simulink library "Computer_Library"  (Simulink 8.1)
settings: Solver=ode45  StartTime=0.0  StopTime=10.0  RelTol=1e-3
values from neighbouring files (symbols this model uses):
  A = 10    [CharTable.m]
  ARROW_DOWN = 48    [CharTable.m]
  ARROW_LEFT = 49    [CharTable.m]
  ARROW_RIGHT = 50    [CharTable.m]
  ARROW_UP = 47    [CharTable.m]
  ASTERISK = 39    [CharTable.m]
  B = 11    [CharTable.m]
  BACKSLASH = 43    [CharTable.m]
  C = 12    [CharTable.m]
  COLON = 40    [CharTable.m]
  COMMA = 53    [CharTable.m]
  CROSS = 38    [CharTable.m]
  CURSOR = 62    [CharTable.m]
  D = 13    [CharTable.m]
  DOT = 52    [CharTable.m]
  EQUAL = 44    [CharTable.m]
  EXCLAMATION_MARK = 55    [CharTable.m]
  F = 15    [CharTable.m]
  G = 16    [CharTable.m]
  GREATER_THAN = 46    [CharTable.m]
  H = 17    [CharTable.m]
  I = 18    [CharTable.m]
  J = 19    [CharTable.m]
  K = 20    [CharTable.m]
  L = 21    [CharTable.m]
  LEFT_PARENTHESES = 59    [CharTable.m]
  LESS_THAN = 45    [CharTable.m]
  M = 22    [CharTable.m]
  MINUS = 37    [CharTable.m]
  N = 23    [CharTable.m]
  O = 24    [CharTable.m]
  P = 25    [CharTable.m]
  PERCENT = 58    [CharTable.m]
  PLUS = 36    [CharTable.m]
  Q = 32    [CharTable.m]
  QUESTION_MARK = 54    [CharTable.m]
  QUOTE = 56    [CharTable.m]
  R = 26    [CharTable.m]
  RECTANGLE = 63    [CharTable.m]
  RIGHT_PARENTHESES = 60    [CharTable.m]
  RomCode = reshape(transpose(RomCode), [], 1)    [ROM.m]
  S = 27    [CharTable.m]
  SEMICOLON = 41    [CharTable.m]
  SHARP = 57    [CharTable.m]
  SLASH = 42    [CharTable.m]
  SPACE = 61    [CharTable.m]
  T = 28    [CharTable.m]
  U = 29    [CharTable.m]
  UNDERSCORE = 51    [CharTable.m]
  V = 30    [CharTable.m]
  W = 31    [CharTable.m]
  X = 33    [CharTable.m]
  Y = 34    [CharTable.m]
  Z = 35    [CharTable.m]
undefined symbols (not defined in the file or in its folder): char_0
libraries: Memory_Blocks_Lib x116, Byte_Multiplexers_Lib x44, commutil2 x18, Bit_Multiplexers_Lib x17, Decoders_Lib x9, simulink_extras x8, Logic_Operations_Lib x4, Byte_Demultiplexers_Lib x2, Arithmetic_Operations_Lib x2, dspsnks4 x1
(part 3 of 4)

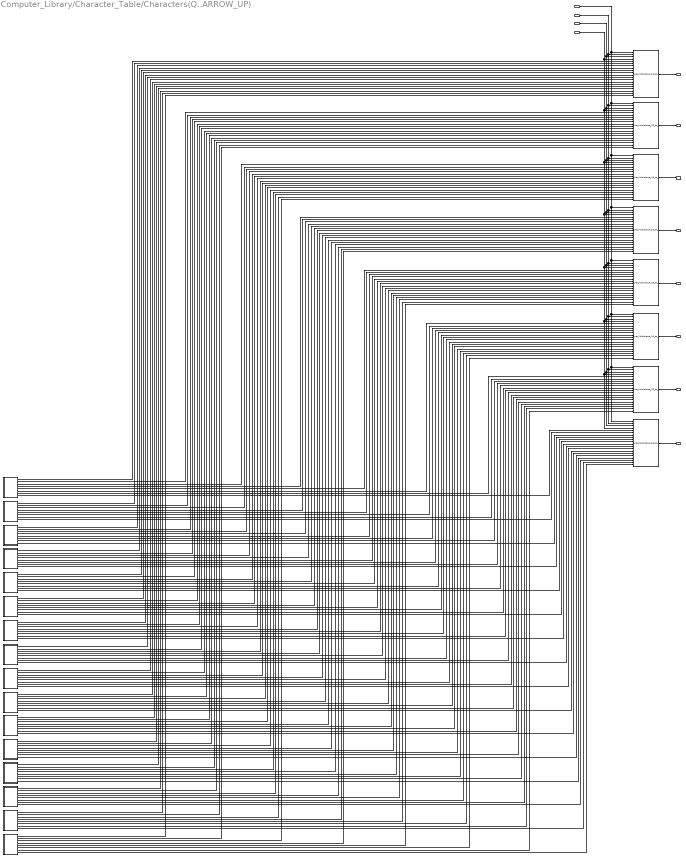
== system Computer_Library/Character_Table/Characters(Q..ARROW_UP) ==
  Address_3_In(1b) : Inport
  Address_2_In(1b) : Inport  Port=2
  Address_1_In(1b) : Inport  Port=3
  Address_0_In(1b) : Inport  Port=4
  16_to_1_Byte_Multiplexer{,1..7} (8 alike) : Byte_Multiplexers_Lib/Byte_Multiplexers_Lib/Byte_Multiplexer_16_to_1
  Char_ARROW_UP : Subsystem
  Char_ASTERISK : Subsystem
  Char_BACKSLASH : Subsystem
  Char_COLON : Subsystem
  Char_CROSS : Subsystem
  Char_EQUAL : Subsystem
  Char_GREATER_THAN : Subsystem
  Char_LESS_THAN : Subsystem
  Char_MINUS : Subsystem
  Char_PLUS : Subsystem
  Char_Q : Subsystem
  Char_SEMICOLON : Subsystem
  Char_SLASH : Subsystem
  Char_X : Subsystem
  Char_Y : Subsystem
  Char_Z : Subsystem
  Column_1(1B) : Outport
  Column_2(1B) : Outport  Port=2
  Column_3(1B) : Outport  Port=3
  Column_4(1B) : Outport  Port=4
  Column_5(1B) : Outport  Port=5
  Column_6(1B) : Outport  Port=6
  Column_7(1B) : Outport  Port=7
  Column_8(1B) : Outport  Port=8
  wires:
  Char_ARROW_UP/1(Column_1(1B)) -> 16_to_1_Byte_Multiplexer/5
  Char_GREATER_THAN/1(Column_1(1B)) -> 16_to_1_Byte_Multiplexer/6
  Char_LESS_THAN/1(Column_1(1B)) -> 16_to_1_Byte_Multiplexer/7
  Char_EQUAL/1(Column_1(1B)) -> 16_to_1_Byte_Multiplexer/8
  Char_BACKSLASH/1(Column_1(1B)) -> 16_to_1_Byte_Multiplexer/9
  Char_SLASH/1(Column_1(1B)) -> 16_to_1_Byte_Multiplexer/10
  Char_SEMICOLON/1(Column_1(1B)) -> 16_to_1_Byte_Multiplexer/11
  Char_COLON/1(Column_1(1B)) -> 16_to_1_Byte_Multiplexer/12
  Char_ASTERISK/1(Column_1(1B)) -> 16_to_1_Byte_Multiplexer/13
  Char_CROSS/1(Column_1(1B)) -> 16_to_1_Byte_Multiplexer/14
  Char_MINUS/1(Column_1(1B)) -> 16_to_1_Byte_Multiplexer/15
  Char_PLUS/1(Column_1(1B)) -> 16_to_1_Byte_Multiplexer/16
  Char_Z/1(Column_1(1B)) -> 16_to_1_Byte_Multiplexer/17
  Char_Y/1(Column_1(1B)) -> 16_to_1_Byte_Multiplexer/18
  Char_X/1(Column_1(1B)) -> 16_to_1_Byte_Multiplexer/19
  Char_Q/1(Column_1(1B)) -> 16_to_1_Byte_Multiplexer/20
  Char_ARROW_UP/2(Column_2(1B)) -> 16_to_1_Byte_Multiplexer1/5
  Char_Q/2(Column_2(1B)) -> 16_to_1_Byte_Multiplexer1/20
  Char_X/2(Column_2(1B)) -> 16_to_1_Byte_Multiplexer1/19
  Char_Y/2(Column_2(1B)) -> 16_to_1_Byte_Multiplexer1/18
  Char_Z/2(Column_2(1B)) -> 16_to_1_Byte_Multiplexer1/17
  Char_PLUS/2(Column_2(1B)) -> 16_to_1_Byte_Multiplexer1/16
  Char_MINUS/2(Column_2(1B)) -> 16_to_1_Byte_Multiplexer1/15
  Char_CROSS/2(Column_2(1B)) -> 16_to_1_Byte_Multiplexer1/14
  Char_ASTERISK/2(Column_2(1B)) -> 16_to_1_Byte_Multiplexer1/13
  Char_COLON/2(Column_2(1B)) -> 16_to_1_Byte_Multiplexer1/12
  Char_SEMICOLON/2(Column_2(1B)) -> 16_to_1_Byte_Multiplexer1/11
  Char_SLASH/2(Column_2(1B)) -> 16_to_1_Byte_Multiplexer1/10
  Char_BACKSLASH/2(Column_2(1B)) -> 16_to_1_Byte_Multiplexer1/9
  Char_EQUAL/2(Column_2(1B)) -> 16_to_1_Byte_Multiplexer1/8
  Char_LESS_THAN/2(Column_2(1B)) -> 16_to_1_Byte_Multiplexer1/7
  Char_GREATER_THAN/2(Column_2(1B)) -> 16_to_1_Byte_Multiplexer1/6
  Char_Q/3(Column_3(1B)) -> 16_to_1_Byte_Multiplexer2/20
  Char_X/3(Column_3(1B)) -> 16_to_1_Byte_Multiplexer2/19
  Char_Y/3(Column_3(1B)) -> 16_to_1_Byte_Multiplexer2/18
  Char_Z/3(Column_3(1B)) -> 16_to_1_Byte_Multiplexer2/17
  Char_PLUS/3(Column_3(1B)) -> 16_to_1_Byte_Multiplexer2/16
  Char_MINUS/3(Column_3(1B)) -> 16_to_1_Byte_Multiplexer2/15
  Char_CROSS/3(Column_3(1B)) -> 16_to_1_Byte_Multiplexer2/14
  Char_ASTERISK/3(Column_3(1B)) -> 16_to_1_Byte_Multiplexer2/13
  Char_COLON/3(Column_3(1B)) -> 16_to_1_Byte_Multiplexer2/12
  Char_SEMICOLON/3(Column_3(1B)) -> 16_to_1_Byte_Multiplexer2/11
  Char_SLASH/3(Column_3(1B)) -> 16_to_1_Byte_Multiplexer2/10
  Char_BACKSLASH/3(Column_3(1B)) -> 16_to_1_Byte_Multiplexer2/9
  Char_EQUAL/3(Column_3(1B)) -> 16_to_1_Byte_Multiplexer2/8
  Char_LESS_THAN/3(Column_3(1B)) -> 16_to_1_Byte_Multiplexer2/7
  Char_GREATER_THAN/3(Column_3(1B)) -> 16_to_1_Byte_Multiplexer2/6
  Char_ARROW_UP/3(Column_3(1B)) -> 16_to_1_Byte_Multiplexer2/5
  Char_Q/4(Column_4(1B)) -> 16_to_1_Byte_Multiplexer3/20
  Char_X/4(Column_4(1B)) -> 16_to_1_Byte_Multiplexer3/19
  Char_Y/4(Column_4(1B)) -> 16_to_1_Byte_Multiplexer3/18
  Char_Z/4(Column_4(1B)) -> 16_to_1_Byte_Multiplexer3/17
  Char_PLUS/4(Column_4(1B)) -> 16_to_1_Byte_Multiplexer3/16
  Char_MINUS/4(Column_4(1B)) -> 16_to_1_Byte_Multiplexer3/15
  Char_CROSS/4(Column_4(1B)) -> 16_to_1_Byte_Multiplexer3/14
  Char_ASTERISK/4(Column_4(1B)) -> 16_to_1_Byte_Multiplexer3/13
  Char_COLON/4(Column_4(1B)) -> 16_to_1_Byte_Multiplexer3/12
  Char_SEMICOLON/4(Column_4(1B)) -> 16_to_1_Byte_Multiplexer3/11
  Char_SLASH/4(Column_4(1B)) -> 16_to_1_Byte_Multiplexer3/10
  Char_BACKSLASH/4(Column_4(1B)) -> 16_to_1_Byte_Multiplexer3/9
  Char_EQUAL/4(Column_4(1B)) -> 16_to_1_Byte_Multiplexer3/8
  Char_LESS_THAN/4(Column_4(1B)) -> 16_to_1_Byte_Multiplexer3/7
  Char_GREATER_THAN/4(Column_4(1B)) -> 16_to_1_Byte_Multiplexer3/6
  Char_ARROW_UP/4(Column_4(1B)) -> 16_to_1_Byte_Multiplexer3/5
  Char_Q/5(Column_5(1B)) -> 16_to_1_Byte_Multiplexer4/20
  Char_X/5(Column_5(1B)) -> 16_to_1_Byte_Multiplexer4/19
  Char_Y/5(Column_5(1B)) -> 16_to_1_Byte_Multiplexer4/18
  Char_Z/5(Column_5(1B)) -> 16_to_1_Byte_Multiplexer4/17
  Char_PLUS/5(Column_5(1B)) -> 16_to_1_Byte_Multiplexer4/16
  Char_MINUS/5(Column_5(1B)) -> 16_to_1_Byte_Multiplexer4/15
  Char_ASTERISK/5(Column_5(1B)) -> 16_to_1_Byte_Multiplexer4/13
  Char_CROSS/5(Column_5(1B)) -> 16_to_1_Byte_Multiplexer4/14
  Char_COLON/5(Column_5(1B)) -> 16_to_1_Byte_Multiplexer4/12
  Char_SEMICOLON/5(Column_5(1B)) -> 16_to_1_Byte_Multiplexer4/11
  Char_SLASH/5(Column_5(1B)) -> 16_to_1_Byte_Multiplexer4/10
  Char_BACKSLASH/5(Column_5(1B)) -> 16_to_1_Byte_Multiplexer4/9
  Char_EQUAL/5(Column_5(1B)) -> 16_to_1_Byte_Multiplexer4/8
  Char_LESS_THAN/5(Column_5(1B)) -> 16_to_1_Byte_Multiplexer4/7
  Char_GREATER_THAN/5(Column_5(1B)) -> 16_to_1_Byte_Multiplexer4/6
  Char_ARROW_UP/5(Column_5(1B)) -> 16_to_1_Byte_Multiplexer4/5
  Char_Q/6(Column_6(1B)) -> 16_to_1_Byte_Multiplexer5/20
  Char_X/6(Column_6(1B)) -> 16_to_1_Byte_Multiplexer5/19
  Char_Y/6(Column_6(1B)) -> 16_to_1_Byte_Multiplexer5/18
  Char_Z/6(Column_6(1B)) -> 16_to_1_Byte_Multiplexer5/17
  Char_PLUS/6(Column_6(1B)) -> 16_to_1_Byte_Multiplexer5/16
  Char_MINUS/6(Column_6(1B)) -> 16_to_1_Byte_Multiplexer5/15
  Char_CROSS/6(Column_6(1B)) -> 16_to_1_Byte_Multiplexer5/14
  Char_ASTERISK/6(Column_6(1B)) -> 16_to_1_Byte_Multiplexer5/13
  Char_COLON/6(Column_6(1B)) -> 16_to_1_Byte_Multiplexer5/12
  Char_SEMICOLON/6(Column_6(1B)) -> 16_to_1_Byte_Multiplexer5/11
  Char_SLASH/6(Column_6(1B)) -> 16_to_1_Byte_Multiplexer5/10
  Char_BACKSLASH/6(Column_6(1B)) -> 16_to_1_Byte_Multiplexer5/9
  Char_EQUAL/7(Column_7(1B)) -> 16_to_1_Byte_Multiplexer6/8
  Char_EQUAL/6(Column_6(1B)) -> 16_to_1_Byte_Multiplexer5/8
  Char_LESS_THAN/6(Column_6(1B)) -> 16_to_1_Byte_Multiplexer5/7
  Char_GREATER_THAN/6(Column_6(1B)) -> 16_to_1_Byte_Multiplexer5/6
  Char_ARROW_UP/6(Column_6(1B)) -> 16_to_1_Byte_Multiplexer5/5
  Char_Q/7(Column_7(1B)) -> 16_to_1_Byte_Multiplexer6/20
  Char_X/7(Column_7(1B)) -> 16_to_1_Byte_Multiplexer6/19
  Char_Y/7(Column_7(1B)) -> 16_to_1_Byte_Multiplexer6/18
  Char_Z/7(Column_7(1B)) -> 16_to_1_Byte_Multiplexer6/17
  Char_PLUS/7(Column_7(1B)) -> 16_to_1_Byte_Multiplexer6/16
  Char_MINUS/7(Column_7(1B)) -> 16_to_1_Byte_Multiplexer6/15
  Char_CROSS/7(Column_7(1B)) -> 16_to_1_Byte_Multiplexer6/14
  Char_ASTERISK/7(Column_7(1B)) -> 16_to_1_Byte_Multiplexer6/13
  Char_COLON/7(Column_7(1B)) -> 16_to_1_Byte_Multiplexer6/12
  Char_SEMICOLON/7(Column_7(1B)) -> 16_to_1_Byte_Multiplexer6/11
  Char_SLASH/7(Column_7(1B)) -> 16_to_1_Byte_Multiplexer6/10
  Char_BACKSLASH/7(Column_7(1B)) -> 16_to_1_Byte_Multiplexer6/9
  Char_LESS_THAN/7(Column_7(1B)) -> 16_to_1_Byte_Multiplexer6/7
  Char_GREATER_THAN/7(Column_7(1B)) -> 16_to_1_Byte_Multiplexer6/6
  Char_ARROW_UP/7(Column_7(1B)) -> 16_to_1_Byte_Multiplexer6/5
  Char_Q/8(Column_8(1B)) -> 16_to_1_Byte_Multiplexer7/20
  Char_X/8(Column_8(1B)) -> 16_to_1_Byte_Multiplexer7/19
  Char_Y/8(Column_8(1B)) -> 16_to_1_Byte_Multiplexer7/18
  Char_Z/8(Column_8(1B)) -> 16_to_1_Byte_Multiplexer7/17
  Char_PLUS/8(Column_8(1B)) -> 16_to_1_Byte_Multiplexer7/16
  Char_MINUS/8(Column_8(1B)) -> 16_to_1_Byte_Multiplexer7/15
  Char_CROSS/8(Column_8(1B)) -> 16_to_1_Byte_Multiplexer7/14
  Char_ASTERISK/8(Column_8(1B)) -> 16_to_1_Byte_Multiplexer7/13
  Char_COLON/8(Column_8(1B)) -> 16_to_1_Byte_Multiplexer7/12
  Char_SEMICOLON/8(Column_8(1B)) -> 16_to_1_Byte_Multiplexer7/11
  Char_SLASH/8(Column_8(1B)) -> 16_to_1_Byte_Multiplexer7/10
  Char_BACKSLASH/8(Column_8(1B)) -> 16_to_1_Byte_Multiplexer7/9
  Char_EQUAL/8(Column_8(1B)) -> 16_to_1_Byte_Multiplexer7/8
  Char_LESS_THAN/8(Column_8(1B)) -> 16_to_1_Byte_Multiplexer7/7
  Char_GREATER_THAN/8(Column_8(1B)) -> 16_to_1_Byte_Multiplexer7/6
  Char_ARROW_UP/8(Column_8(1B)) -> 16_to_1_Byte_Multiplexer7/5
  16_to_1_Byte_Multiplexer/1 -> Column_1(1B)/1
  16_to_1_Byte_Multiplexer1/1 -> Column_2(1B)/1
  16_to_1_Byte_Multiplexer2/1 -> Column_3(1B)/1
  16_to_1_Byte_Multiplexer3/1 -> Column_4(1B)/1
  16_to_1_Byte_Multiplexer4/1 -> Column_5(1B)/1
  16_to_1_Byte_Multiplexer5/1 -> Column_6(1B)/1
  16_to_1_Byte_Multiplexer6/1 -> Column_7(1B)/1
  16_to_1_Byte_Multiplexer7/1 -> Column_8(1B)/1
  Address_0_In(1b)/1 -> 16_to_1_Byte_Multiplexer/4, 16_to_1_Byte_Multiplexer1/4, 16_to_1_Byte_Multiplexer2/4, 16_to_1_Byte_Multiplexer3/4, 16_to_1_Byte_Multiplexer4/4, 16_to_1_Byte_Multiplexer5/4, 16_to_1_Byte_Multiplexer6/4, 16_to_1_Byte_Multiplexer7/4
  Address_1_In(1b)/1 -> 16_to_1_Byte_Multiplexer/3, 16_to_1_Byte_Multiplexer1/3, 16_to_1_Byte_Multiplexer2/3, 16_to_1_Byte_Multiplexer3/3, 16_to_1_Byte_Multiplexer4/3, 16_to_1_Byte_Multiplexer5/3, 16_to_1_Byte_Multiplexer6/3, 16_to_1_Byte_Multiplexer7/3
  Address_2_In(1b)/1 -> 16_to_1_Byte_Multiplexer/2, 16_to_1_Byte_Multiplexer1/2, 16_to_1_Byte_Multiplexer2/2, 16_to_1_Byte_Multiplexer3/2, 16_to_1_Byte_Multiplexer4/2, 16_to_1_Byte_Multiplexer5/2, 16_to_1_Byte_Multiplexer6/2, 16_to_1_Byte_Multiplexer7/2
  Address_3_In(1b)/1 -> 16_to_1_Byte_Multiplexer/1, 16_to_1_Byte_Multiplexer1/1, 16_to_1_Byte_Multiplexer2/1, 16_to_1_Byte_Multiplexer3/1, 16_to_1_Byte_Multiplexer4/1, 16_to_1_Byte_Multiplexer5/1, 16_to_1_Byte_Multiplexer6/1, 16_to_1_Byte_Multiplexer7/1

== system Computer_Library/Instruction_ADD/Full_Adder ==
  A : Inport
  B : Inport  Port=2
  Carry_In : Inport  Port=3
  Logical Operator : Logic  Operator=XOR  IconShape=distinctive  AllPortsSameDT=off  OutDataTypeStr=boolean
  Logical Operator1 : Logic  IconShape=distinctive  AllPortsSameDT=off  OutDataTypeStr=boolean
  Logical Operator2 : Logic  Operator=XOR  IconShape=distinctive  AllPortsSameDT=off  OutDataTypeStr=boolean
  Logical Operator3 : Logic  IconShape=distinctive  AllPortsSameDT=off  OutDataTypeStr=boolean
  Logical Operator4 : Logic  Operator=OR  IconShape=distinctive  AllPortsSameDT=off  OutDataTypeStr=boolean
  Carry_Out : Outport
  Sum : Outport  Port=2
  wires:
  A/1 -> Logical Operator1/1, Logical Operator/1
  B/1 -> Logical Operator1/2, Logical Operator/2
  Logical Operator2/1 -> Sum/1
  Logical Operator/1 -> Logical Operator3/1, Logical Operator2/1
  Carry_In/1 -> Logical Operator2/2, Logical Operator3/2
  Logical Operator3/1 -> Logical Operator4/1
  Logical Operator1/1 -> Logical Operator4/2
  Logical Operator4/1 -> Carry_Out/1

== system Computer_Library/Instruction_ADD/Full_Adder1 ==
  A : Inport
  B : Inport  Port=2
  Carry_In : Inport  Port=3
  Logical Operator : Logic  Operator=XOR  IconShape=distinctive  AllPortsSameDT=off  OutDataTypeStr=boolean
  Logical Operator1 : Logic  IconShape=distinctive  AllPortsSameDT=off  OutDataTypeStr=boolean
  Logical Operator2 : Logic  Operator=XOR  IconShape=distinctive  AllPortsSameDT=off  OutDataTypeStr=boolean
  Logical Operator3 : Logic  IconShape=distinctive  AllPortsSameDT=off  OutDataTypeStr=boolean
  Logical Operator4 : Logic  Operator=OR  IconShape=distinctive  AllPortsSameDT=off  OutDataTypeStr=boolean
  Carry_Out : Outport
  Sum : Outport  Port=2
  wires:
  A/1 -> Logical Operator1/1, Logical Operator/1
  B/1 -> Logical Operator1/2, Logical Operator/2
  Logical Operator2/1 -> Sum/1
  Logical Operator/1 -> Logical Operator3/1, Logical Operator2/1
  Carry_In/1 -> Logical Operator2/2, Logical Operator3/2
  Logical Operator3/1 -> Logical Operator4/1
  Logical Operator1/1 -> Logical Operator4/2
  Logical Operator4/1 -> Carry_Out/1

== system Computer_Library/Instruction_ADD/Full_Adder2 ==
  A : Inport
  B : Inport  Port=2
  Carry_In : Inport  Port=3
  Logical Operator : Logic  Operator=XOR  IconShape=distinctive  AllPortsSameDT=off  OutDataTypeStr=boolean
  Logical Operator1 : Logic  IconShape=distinctive  AllPortsSameDT=off  OutDataTypeStr=boolean
  Logical Operator2 : Logic  Operator=XOR  IconShape=distinctive  AllPortsSameDT=off  OutDataTypeStr=boolean
  Logical Operator3 : Logic  IconShape=distinctive  AllPortsSameDT=off  OutDataTypeStr=boolean
  Logical Operator4 : Logic  Operator=OR  IconShape=distinctive  AllPortsSameDT=off  OutDataTypeStr=boolean
  Carry_Out : Outport
  Sum : Outport  Port=2
  wires:
  A/1 -> Logical Operator1/1, Logical Operator/1
  B/1 -> Logical Operator1/2, Logical Operator/2
  Logical Operator2/1 -> Sum/1
  Logical Operator/1 -> Logical Operator3/1, Logical Operator2/1
  Carry_In/1 -> Logical Operator2/2, Logical Operator3/2
  Logical Operator3/1 -> Logical Operator4/1
  Logical Operator1/1 -> Logical Operator4/2
  Logical Operator4/1 -> Carry_Out/1

== system Computer_Library/Instruction_ADD/Full_Adder3 ==
  A : Inport
  B : Inport  Port=2
  Carry_In : Inport  Port=3
  Logical Operator : Logic  Operator=XOR  IconShape=distinctive  AllPortsSameDT=off  OutDataTypeStr=boolean
  Logical Operator1 : Logic  IconShape=distinctive  AllPortsSameDT=off  OutDataTypeStr=boolean
  Logical Operator2 : Logic  Operator=XOR  IconShape=distinctive  AllPortsSameDT=off  OutDataTypeStr=boolean
  Logical Operator3 : Logic  IconShape=distinctive  AllPortsSameDT=off  OutDataTypeStr=boolean
  Logical Operator4 : Logic  Operator=OR  IconShape=distinctive  AllPortsSameDT=off  OutDataTypeStr=boolean
  Carry_Out : Outport
  Sum : Outport  Port=2
  wires:
  A/1 -> Logical Operator1/1, Logical Operator/1
  B/1 -> Logical Operator1/2, Logical Operator/2
  Logical Operator2/1 -> Sum/1
  Logical Operator/1 -> Logical Operator3/1, Logical Operator2/1
  Carry_In/1 -> Logical Operator2/2, Logical Operator3/2
  Logical Operator3/1 -> Logical Operator4/1
  Logical Operator1/1 -> Logical Operator4/2
  Logical Operator4/1 -> Carry_Out/1

== system Computer_Library/Instruction_ADD/Full_Adder4 ==
  A : Inport
  B : Inport  Port=2
  Carry_In : Inport  Port=3
  Logical Operator : Logic  Operator=XOR  IconShape=distinctive  AllPortsSameDT=off  OutDataTypeStr=boolean
  Logical Operator1 : Logic  IconShape=distinctive  AllPortsSameDT=off  OutDataTypeStr=boolean
  Logical Operator2 : Logic  Operator=XOR  IconShape=distinctive  AllPortsSameDT=off  OutDataTypeStr=boolean
  Logical Operator3 : Logic  IconShape=distinctive  AllPortsSameDT=off  OutDataTypeStr=boolean
  Logical Operator4 : Logic  Operator=OR  IconShape=distinctive  AllPortsSameDT=off  OutDataTypeStr=boolean
  Carry_Out : Outport
  Sum : Outport  Port=2
  wires:
  A/1 -> Logical Operator1/1, Logical Operator/1
  B/1 -> Logical Operator1/2, Logical Operator/2
  Logical Operator2/1 -> Sum/1
  Logical Operator/1 -> Logical Operator3/1, Logical Operator2/1
  Carry_In/1 -> Logical Operator2/2, Logical Operator3/2
  Logical Operator3/1 -> Logical Operator4/1
  Logical Operator1/1 -> Logical Operator4/2
  Logical Operator4/1 -> Carry_Out/1

== system Computer_Library/Instruction_ADD/Full_Adder5 ==
  A : Inport
  B : Inport  Port=2
  Carry_In : Inport  Port=3
  Logical Operator : Logic  Operator=XOR  IconShape=distinctive  AllPortsSameDT=off  OutDataTypeStr=boolean
  Logical Operator1 : Logic  IconShape=distinctive  AllPortsSameDT=off  OutDataTypeStr=boolean
  Logical Operator2 : Logic  Operator=XOR  IconShape=distinctive  AllPortsSameDT=off  OutDataTypeStr=boolean
  Logical Operator3 : Logic  IconShape=distinctive  AllPortsSameDT=off  OutDataTypeStr=boolean
  Logical Operator4 : Logic  Operator=OR  IconShape=distinctive  AllPortsSameDT=off  OutDataTypeStr=boolean
  Carry_Out : Outport
  Sum : Outport  Port=2
  wires:
  A/1 -> Logical Operator1/1, Logical Operator/1
  B/1 -> Logical Operator1/2, Logical Operator/2
  Logical Operator2/1 -> Sum/1
  Logical Operator/1 -> Logical Operator3/1, Logical Operator2/1
  Carry_In/1 -> Logical Operator2/2, Logical Operator3/2
  Logical Operator3/1 -> Logical Operator4/1
  Logical Operator1/1 -> Logical Operator4/2
  Logical Operator4/1 -> Carry_Out/1

== system Computer_Library/Instruction_ADD/Full_Adder6 ==
  A : Inport
  B : Inport  Port=2
  Carry_In : Inport  Port=3
  Logical Operator : Logic  Operator=XOR  IconShape=distinctive  AllPortsSameDT=off  OutDataTypeStr=boolean
  Logical Operator1 : Logic  IconShape=distinctive  AllPortsSameDT=off  OutDataTypeStr=boolean
  Logical Operator2 : Logic  Operator=XOR  IconShape=distinctive  AllPortsSameDT=off  OutDataTypeStr=boolean
  Logical Operator3 : Logic  IconShape=distinctive  AllPortsSameDT=off  OutDataTypeStr=boolean
  Logical Operator4 : Logic  Operator=OR  IconShape=distinctive  AllPortsSameDT=off  OutDataTypeStr=boolean
  Carry_Out : Outport
  Sum : Outport  Port=2
  wires:
  A/1 -> Logical Operator1/1, Logical Operator/1
  B/1 -> Logical Operator1/2, Logical Operator/2
  Logical Operator2/1 -> Sum/1
  Logical Operator/1 -> Logical Operator3/1, Logical Operator2/1
  Carry_In/1 -> Logical Operator2/2, Logical Operator3/2
  Logical Operator3/1 -> Logical Operator4/1
  Logical Operator1/1 -> Logical Operator4/2
  Logical Operator4/1 -> Carry_Out/1

== system Computer_Library/Instruction_ADD/Full_Adder7 ==
  A : Inport
  B : Inport  Port=2
  Carry_In : Inport  Port=3
  Logical Operator : Logic  Operator=XOR  IconShape=distinctive  AllPortsSameDT=off  OutDataTypeStr=boolean
  Logical Operator1 : Logic  IconShape=distinctive  AllPortsSameDT=off  OutDataTypeStr=boolean
  Logical Operator2 : Logic  Operator=XOR  IconShape=distinctive  AllPortsSameDT=off  OutDataTypeStr=boolean
  Logical Operator3 : Logic  IconShape=distinctive  AllPortsSameDT=off  OutDataTypeStr=boolean
  Logical Operator4 : Logic  Operator=OR  IconShape=distinctive  AllPortsSameDT=off  OutDataTypeStr=boolean
  Carry_Out : Outport
  Sum : Outport  Port=2
  wires:
  A/1 -> Logical Operator1/1, Logical Operator/1
  B/1 -> Logical Operator1/2, Logical Operator/2
  Logical Operator2/1 -> Sum/1
  Logical Operator/1 -> Logical Operator3/1, Logical Operator2/1
  Carry_In/1 -> Logical Operator2/2, Logical Operator3/2
  Logical Operator3/1 -> Logical Operator4/1
  Logical Operator1/1 -> Logical Operator4/2
  Logical Operator4/1 -> Carry_Out/1

== system Computer_Library/Character_Table/Characters(0..F)/Char_0 ==
  Byte_01 : Constant  Value=char_0(:, 2)  OutDataTypeStr=uint8
  Byte_02 : Constant  Value=char_0(:, 3)  OutDataTypeStr=uint8
  Byte_03 : Constant  Value=char_0(:, 4)  OutDataTypeStr=uint8
  Byte_04 : Constant  Value=char_0(:, 5)  OutDataTypeStr=uint8
  Byte_05 : Constant  Value=char_0(:, 6)  OutDataTypeStr=uint8
  Byte_06 : Constant  Value=char_0(:, 7)  OutDataTypeStr=uint8
  Byte_07 : Constant  Value=char_0(:, 8)  OutDataTypeStr=uint8
  Byte_1 : Constant  Value=char_0(:, 1)  OutDataTypeStr=uint8
  Column_1(1B) : Outport
  Column_2(1B) : Outport  Port=2
  Column_3(1B) : Outport  Port=3
  Column_4(1B) : Outport  Port=4
  Column_5(1B) : Outport  Port=5
  Column_6(1B) : Outport  Port=6
  Column_7(1B) : Outport  Port=7
  Column_8(1B) : Outport  Port=8
  wires:
  Byte_05/1 -> Column_6(1B)/1
  Byte_04/1 -> Column_5(1B)/1
  Byte_01/1 -> Column_2(1B)/1
  Byte_07/1 -> Column_8(1B)/1
  Byte_03/1 -> Column_4(1B)/1
  Byte_06/1 -> Column_7(1B)/1
  Byte_1/1 -> Column_1(1B)/1
  Byte_02/1 -> Column_3(1B)/1

== system Computer_Library/Character_Table/Characters(0..F)/Char_1 ==
  Byte_01 : Constant  Value=char(2, 1)  OutDataTypeStr=uint8
  Byte_02 : Constant  Value=char(3, 1)  OutDataTypeStr=uint8
  Byte_03 : Constant  Value=char(4, 1)  OutDataTypeStr=uint8
  Byte_04 : Constant  Value=char(5, 1)  OutDataTypeStr=uint8
  Byte_05 : Constant  Value=char(6, 1)  OutDataTypeStr=uint8
  Byte_06 : Constant  Value=char(7, 1)  OutDataTypeStr=uint8
  Byte_07 : Constant  Value=char(8, 1)  OutDataTypeStr=uint8
  Byte_1 : Constant  Value=char(1, 1)  OutDataTypeStr=uint8
  Column_1(1B) : Outport
  Column_2(1B) : Outport  Port=2
  Column_3(1B) : Outport  Port=3
  Column_4(1B) : Outport  Port=4
  Column_5(1B) : Outport  Port=5
  Column_6(1B) : Outport  Port=6
  Column_7(1B) : Outport  Port=7
  Column_8(1B) : Outport  Port=8
  wires:
  Byte_05/1 -> Column_6(1B)/1
  Byte_04/1 -> Column_5(1B)/1
  Byte_01/1 -> Column_2(1B)/1
  Byte_07/1 -> Column_8(1B)/1
  Byte_03/1 -> Column_4(1B)/1
  Byte_06/1 -> Column_7(1B)/1
  Byte_1/1 -> Column_1(1B)/1
  Byte_02/1 -> Column_3(1B)/1

== system Computer_Library/Character_Table/Characters(0..F)/Char_2 ==
  Byte_01 : Constant  Value=char(2, 2)  OutDataTypeStr=uint8
  Byte_02 : Constant  Value=char(3, 2)  OutDataTypeStr=uint8
  Byte_03 : Constant  Value=char(4, 2)  OutDataTypeStr=uint8
  Byte_04 : Constant  Value=char(5, 2)  OutDataTypeStr=uint8
  Byte_05 : Constant  Value=char(6, 2)  OutDataTypeStr=uint8
  Byte_06 : Constant  Value=char(7, 2)  OutDataTypeStr=uint8
  Byte_07 : Constant  Value=char(8, 2)  OutDataTypeStr=uint8
  Byte_1 : Constant  Value=char(1, 2)  OutDataTypeStr=uint8
  Column_1(1B) : Outport
  Column_2(1B) : Outport  Port=2
  Column_3(1B) : Outport  Port=3
  Column_4(1B) : Outport  Port=4
  Column_5(1B) : Outport  Port=5
  Column_6(1B) : Outport  Port=6
  Column_7(1B) : Outport  Port=7
  Column_8(1B) : Outport  Port=8
  wires:
  Byte_05/1 -> Column_6(1B)/1
  Byte_04/1 -> Column_5(1B)/1
  Byte_01/1 -> Column_2(1B)/1
  Byte_07/1 -> Column_8(1B)/1
  Byte_03/1 -> Column_4(1B)/1
  Byte_06/1 -> Column_7(1B)/1
  Byte_1/1 -> Column_1(1B)/1
  Byte_02/1 -> Column_3(1B)/1

== system Computer_Library/Character_Table/Characters(0..F)/Char_3 ==
  Byte_01 : Constant  Value=char(2, 3)  OutDataTypeStr=uint8
  Byte_02 : Constant  Value=char(3, 3)  OutDataTypeStr=uint8
  Byte_03 : Constant  Value=char(4, 3)  OutDataTypeStr=uint8
  Byte_04 : Constant  Value=char(5, 3)  OutDataTypeStr=uint8
  Byte_05 : Constant  Value=char(6, 3)  OutDataTypeStr=uint8
  Byte_06 : Constant  Value=char(7, 3)  OutDataTypeStr=uint8
  Byte_07 : Constant  Value=char(8, 3)  OutDataTypeStr=uint8
  Byte_1 : Constant  Value=char(1, 3)  OutDataTypeStr=uint8
  Column_1(1B) : Outport
  Column_2(1B) : Outport  Port=2
  Column_3(1B) : Outport  Port=3
  Column_4(1B) : Outport  Port=4
  Column_5(1B) : Outport  Port=5
  Column_6(1B) : Outport  Port=6
  Column_7(1B) : Outport  Port=7
  Column_8(1B) : Outport  Port=8
  wires:
  Byte_05/1 -> Column_6(1B)/1
  Byte_04/1 -> Column_5(1B)/1
  Byte_01/1 -> Column_2(1B)/1
  Byte_07/1 -> Column_8(1B)/1
  Byte_03/1 -> Column_4(1B)/1
  Byte_06/1 -> Column_7(1B)/1
  Byte_1/1 -> Column_1(1B)/1
  Byte_02/1 -> Column_3(1B)/1

== system Computer_Library/Character_Table/Characters(0..F)/Char_4 ==
  Byte_01 : Constant  Value=char(2, 4)  OutDataTypeStr=uint8
  Byte_02 : Constant  Value=char(3, 4)  OutDataTypeStr=uint8
  Byte_03 : Constant  Value=char(4, 4)  OutDataTypeStr=uint8
  Byte_04 : Constant  Value=char(5, 4)  OutDataTypeStr=uint8
  Byte_05 : Constant  Value=char(6, 4)  OutDataTypeStr=uint8
  Byte_06 : Constant  Value=char(7, 4)  OutDataTypeStr=uint8
  Byte_07 : Constant  Value=char(8, 4)  OutDataTypeStr=uint8
  Byte_1 : Constant  Value=char(1, 4)  OutDataTypeStr=uint8
  Column_1(1B) : Outport
  Column_2(1B) : Outport  Port=2
  Column_3(1B) : Outport  Port=3
  Column_4(1B) : Outport  Port=4
  Column_5(1B) : Outport  Port=5
  Column_6(1B) : Outport  Port=6
  Column_7(1B) : Outport  Port=7
  Column_8(1B) : Outport  Port=8
  wires:
  Byte_05/1 -> Column_6(1B)/1
  Byte_04/1 -> Column_5(1B)/1
  Byte_01/1 -> Column_2(1B)/1
  Byte_07/1 -> Column_8(1B)/1
  Byte_03/1 -> Column_4(1B)/1
  Byte_06/1 -> Column_7(1B)/1
  Byte_1/1 -> Column_1(1B)/1
  Byte_02/1 -> Column_3(1B)/1

== system Computer_Library/Character_Table/Characters(0..F)/Char_5 ==
  Byte_01 : Constant  Value=char(2, 5)  OutDataTypeStr=uint8
  Byte_02 : Constant  Value=char(3, 5)  OutDataTypeStr=uint8
  Byte_03 : Constant  Value=char(4, 5)  OutDataTypeStr=uint8
  Byte_04 : Constant  Value=char(5, 5)  OutDataTypeStr=uint8
  Byte_05 : Constant  Value=char(6, 5)  OutDataTypeStr=uint8
  Byte_06 : Constant  Value=char(7, 5)  OutDataTypeStr=uint8
  Byte_07 : Constant  Value=char(8, 5)  OutDataTypeStr=uint8
  Byte_1 : Constant  Value=char(1, 5)  OutDataTypeStr=uint8
  Column_1(1B) : Outport
  Column_2(1B) : Outport  Port=2
  Column_3(1B) : Outport  Port=3
  Column_4(1B) : Outport  Port=4
  Column_5(1B) : Outport  Port=5
  Column_6(1B) : Outport  Port=6
  Column_7(1B) : Outport  Port=7
  Column_8(1B) : Outport  Port=8
  wires:
  Byte_05/1 -> Column_6(1B)/1
  Byte_04/1 -> Column_5(1B)/1
  Byte_01/1 -> Column_2(1B)/1
  Byte_07/1 -> Column_8(1B)/1
  Byte_03/1 -> Column_4(1B)/1
  Byte_06/1 -> Column_7(1B)/1
  Byte_1/1 -> Column_1(1B)/1
  Byte_02/1 -> Column_3(1B)/1

== system Computer_Library/Character_Table/Characters(0..F)/Char_6 ==
  Byte_01 : Constant  Value=char(2, 6)  OutDataTypeStr=uint8
  Byte_02 : Constant  Value=char(3, 6)  OutDataTypeStr=uint8
  Byte_03 : Constant  Value=char(4, 6)  OutDataTypeStr=uint8
  Byte_04 : Constant  Value=char(5, 6)  OutDataTypeStr=uint8
  Byte_05 : Constant  Value=char(6, 6)  OutDataTypeStr=uint8
  Byte_06 : Constant  Value=char(7, 6)  OutDataTypeStr=uint8
  Byte_07 : Constant  Value=char(8, 6)  OutDataTypeStr=uint8
  Byte_1 : Constant  Value=char(1, 6)  OutDataTypeStr=uint8
  Column_1(1B) : Outport
  Column_2(1B) : Outport  Port=2
  Column_3(1B) : Outport  Port=3
  Column_4(1B) : Outport  Port=4
  Column_5(1B) : Outport  Port=5
  Column_6(1B) : Outport  Port=6
  Column_7(1B) : Outport  Port=7
  Column_8(1B) : Outport  Port=8
  wires:
  Byte_05/1 -> Column_6(1B)/1
  Byte_04/1 -> Column_5(1B)/1
  Byte_01/1 -> Column_2(1B)/1
  Byte_07/1 -> Column_8(1B)/1
  Byte_03/1 -> Column_4(1B)/1
  Byte_06/1 -> Column_7(1B)/1
  Byte_1/1 -> Column_1(1B)/1
  Byte_02/1 -> Column_3(1B)/1

== system Computer_Library/Character_Table/Characters(0..F)/Char_7 ==
  Byte_01 : Constant  Value=char(2, 7)  OutDataTypeStr=uint8
  Byte_02 : Constant  Value=char(3, 7)  OutDataTypeStr=uint8
  Byte_03 : Constant  Value=char(4, 7)  OutDataTypeStr=uint8
  Byte_04 : Constant  Value=char(5, 7)  OutDataTypeStr=uint8
  Byte_05 : Constant  Value=char(6, 7)  OutDataTypeStr=uint8
  Byte_06 : Constant  Value=char(7, 7)  OutDataTypeStr=uint8
  Byte_07 : Constant  Value=char(8, 7)  OutDataTypeStr=uint8
  Byte_1 : Constant  Value=char(1, 7)  OutDataTypeStr=uint8
  Column_1(1B) : Outport
  Column_2(1B) : Outport  Port=2
  Column_3(1B) : Outport  Port=3
  Column_4(1B) : Outport  Port=4
  Column_5(1B) : Outport  Port=5
  Column_6(1B) : Outport  Port=6
  Column_7(1B) : Outport  Port=7
  Column_8(1B) : Outport  Port=8
  wires:
  Byte_05/1 -> Column_6(1B)/1
  Byte_04/1 -> Column_5(1B)/1
  Byte_01/1 -> Column_2(1B)/1
  Byte_07/1 -> Column_8(1B)/1
  Byte_03/1 -> Column_4(1B)/1
  Byte_06/1 -> Column_7(1B)/1
  Byte_1/1 -> Column_1(1B)/1
  Byte_02/1 -> Column_3(1B)/1

== system Computer_Library/Character_Table/Characters(0..F)/Char_8 ==
  Byte_01 : Constant  Value=char(2, 8)  OutDataTypeStr=uint8
  Byte_02 : Constant  Value=char(3, 8)  OutDataTypeStr=uint8
  Byte_03 : Constant  Value=char(4, 8)  OutDataTypeStr=uint8
  Byte_04 : Constant  Value=char(5, 8)  OutDataTypeStr=uint8
  Byte_05 : Constant  Value=char(6, 8)  OutDataTypeStr=uint8
  Byte_06 : Constant  Value=char(7, 8)  OutDataTypeStr=uint8
  Byte_07 : Constant  Value=char(8, 8)  OutDataTypeStr=uint8
  Byte_1 : Constant  Value=char(1, 8)  OutDataTypeStr=uint8
  Column_1(1B) : Outport
  Column_2(1B) : Outport  Port=2
  Column_3(1B) : Outport  Port=3
  Column_4(1B) : Outport  Port=4
  Column_5(1B) : Outport  Port=5
  Column_6(1B) : Outport  Port=6
  Column_7(1B) : Outport  Port=7
  Column_8(1B) : Outport  Port=8
  wires:
  Byte_05/1 -> Column_6(1B)/1
  Byte_04/1 -> Column_5(1B)/1
  Byte_01/1 -> Column_2(1B)/1
  Byte_07/1 -> Column_8(1B)/1
  Byte_03/1 -> Column_4(1B)/1
  Byte_06/1 -> Column_7(1B)/1
  Byte_1/1 -> Column_1(1B)/1
  Byte_02/1 -> Column_3(1B)/1

== system Computer_Library/Character_Table/Characters(0..F)/Char_9 ==
  Byte_01 : Constant  Value=char(2, 9)  OutDataTypeStr=uint8
  Byte_02 : Constant  Value=char(3, 9)  OutDataTypeStr=uint8
  Byte_03 : Constant  Value=char(4, 9)  OutDataTypeStr=uint8
  Byte_04 : Constant  Value=char(5, 9)  OutDataTypeStr=uint8
  Byte_05 : Constant  Value=char(6, 9)  OutDataTypeStr=uint8
  Byte_06 : Constant  Value=char(7, 9)  OutDataTypeStr=uint8
  Byte_07 : Constant  Value=char(8, 9)  OutDataTypeStr=uint8
  Byte_1 : Constant  Value=char(1, 9)  OutDataTypeStr=uint8
  Column_1(1B) : Outport
  Column_2(1B) : Outport  Port=2
  Column_3(1B) : Outport  Port=3
  Column_4(1B) : Outport  Port=4
  Column_5(1B) : Outport  Port=5
  Column_6(1B) : Outport  Port=6
  Column_7(1B) : Outport  Port=7
  Column_8(1B) : Outport  Port=8
  wires:
  Byte_05/1 -> Column_6(1B)/1
  Byte_04/1 -> Column_5(1B)/1
  Byte_01/1 -> Column_2(1B)/1
  Byte_07/1 -> Column_8(1B)/1
  Byte_03/1 -> Column_4(1B)/1
  Byte_06/1 -> Column_7(1B)/1
  Byte_1/1 -> Column_1(1B)/1
  Byte_02/1 -> Column_3(1B)/1

== system Computer_Library/Character_Table/Characters(0..F)/Char_A ==
  Byte_01 : Constant  Value=char(2, A)  OutDataTypeStr=uint8
  Byte_02 : Constant  Value=char(3, A)  OutDataTypeStr=uint8
  Byte_03 : Constant  Value=char(4, A)  OutDataTypeStr=uint8
  Byte_04 : Constant  Value=char(5, A)  OutDataTypeStr=uint8
  Byte_05 : Constant  Value=char(6, A)  OutDataTypeStr=uint8
  Byte_06 : Constant  Value=char(7, A)  OutDataTypeStr=uint8
  Byte_07 : Constant  Value=char(8, A)  OutDataTypeStr=uint8
  Byte_1 : Constant  Value=char(1, A)  OutDataTypeStr=uint8
  Column_1(1B) : Outport
  Column_2(1B) : Outport  Port=2
  Column_3(1B) : Outport  Port=3
  Column_4(1B) : Outport  Port=4
  Column_5(1B) : Outport  Port=5
  Column_6(1B) : Outport  Port=6
  Column_7(1B) : Outport  Port=7
  Column_8(1B) : Outport  Port=8
  wires:
  Byte_05/1 -> Column_6(1B)/1
  Byte_04/1 -> Column_5(1B)/1
  Byte_01/1 -> Column_2(1B)/1
  Byte_07/1 -> Column_8(1B)/1
  Byte_03/1 -> Column_4(1B)/1
  Byte_06/1 -> Column_7(1B)/1
  Byte_1/1 -> Column_1(1B)/1
  Byte_02/1 -> Column_3(1B)/1

== system Computer_Library/Character_Table/Characters(0..F)/Char_B ==
  Byte_01 : Constant  Value=char(2, B)  OutDataTypeStr=uint8
  Byte_02 : Constant  Value=char(3, B)  OutDataTypeStr=uint8
  Byte_03 : Constant  Value=char(4, B)  OutDataTypeStr=uint8
  Byte_04 : Constant  Value=char(5, B)  OutDataTypeStr=uint8
  Byte_05 : Constant  Value=char(6, B)  OutDataTypeStr=uint8
  Byte_06 : Constant  Value=char(7, B)  OutDataTypeStr=uint8
  Byte_07 : Constant  Value=char(8, B)  OutDataTypeStr=uint8
  Byte_1 : Constant  Value=char(1, B)  OutDataTypeStr=uint8
  Column_1(1B) : Outport
  Column_2(1B) : Outport  Port=2
  Column_3(1B) : Outport  Port=3
  Column_4(1B) : Outport  Port=4
  Column_5(1B) : Outport  Port=5
  Column_6(1B) : Outport  Port=6
  Column_7(1B) : Outport  Port=7
  Column_8(1B) : Outport  Port=8
  wires:
  Byte_05/1 -> Column_6(1B)/1
  Byte_04/1 -> Column_5(1B)/1
  Byte_01/1 -> Column_2(1B)/1
  Byte_07/1 -> Column_8(1B)/1
  Byte_03/1 -> Column_4(1B)/1
  Byte_06/1 -> Column_7(1B)/1
  Byte_1/1 -> Column_1(1B)/1
  Byte_02/1 -> Column_3(1B)/1

== system Computer_Library/Character_Table/Characters(0..F)/Char_C ==
  Byte_01 : Constant  Value=char(2, C)  OutDataTypeStr=uint8
  Byte_02 : Constant  Value=char(3, C)  OutDataTypeStr=uint8
  Byte_03 : Constant  Value=char(4, C)  OutDataTypeStr=uint8
  Byte_04 : Constant  Value=char(5, C)  OutDataTypeStr=uint8
  Byte_05 : Constant  Value=char(6, C)  OutDataTypeStr=uint8
  Byte_06 : Constant  Value=char(7, C)  OutDataTypeStr=uint8
  Byte_07 : Constant  Value=char(8, C)  OutDataTypeStr=uint8
  Byte_1 : Constant  Value=char(1, C)  OutDataTypeStr=uint8
  Column_1(1B) : Outport
  Column_2(1B) : Outport  Port=2
  Column_3(1B) : Outport  Port=3
  Column_4(1B) : Outport  Port=4
  Column_5(1B) : Outport  Port=5
  Column_6(1B) : Outport  Port=6
  Column_7(1B) : Outport  Port=7
  Column_8(1B) : Outport  Port=8
  wires:
  Byte_05/1 -> Column_6(1B)/1
  Byte_04/1 -> Column_5(1B)/1
  Byte_01/1 -> Column_2(1B)/1
  Byte_07/1 -> Column_8(1B)/1
  Byte_03/1 -> Column_4(1B)/1
  Byte_06/1 -> Column_7(1B)/1
  Byte_1/1 -> Column_1(1B)/1
  Byte_02/1 -> Column_3(1B)/1

== system Computer_Library/Character_Table/Characters(0..F)/Char_D ==
  Byte_01 : Constant  Value=char(2, D)  OutDataTypeStr=uint8
  Byte_02 : Constant  Value=char(3, D)  OutDataTypeStr=uint8
  Byte_03 : Constant  Value=char(4, D)  OutDataTypeStr=uint8
  Byte_04 : Constant  Value=char(5, D)  OutDataTypeStr=uint8
  Byte_05 : Constant  Value=char(6, D)  OutDataTypeStr=uint8
  Byte_06 : Constant  Value=char(7, D)  OutDataTypeStr=uint8
  Byte_07 : Constant  Value=char(8, D)  OutDataTypeStr=uint8
  Byte_1 : Constant  Value=char(1, D)  OutDataTypeStr=uint8
  Column_1(1B) : Outport
  Column_2(1B) : Outport  Port=2
  Column_3(1B) : Outport  Port=3
  Column_4(1B) : Outport  Port=4
  Column_5(1B) : Outport  Port=5
  Column_6(1B) : Outport  Port=6
  Column_7(1B) : Outport  Port=7
  Column_8(1B) : Outport  Port=8
  wires:
  Byte_05/1 -> Column_6(1B)/1
  Byte_04/1 -> Column_5(1B)/1
  Byte_01/1 -> Column_2(1B)/1
  Byte_07/1 -> Column_8(1B)/1
  Byte_03/1 -> Column_4(1B)/1
  Byte_06/1 -> Column_7(1B)/1
  Byte_1/1 -> Column_1(1B)/1
  Byte_02/1 -> Column_3(1B)/1

== system Computer_Library/Character_Table/Characters(0..F)/Char_E ==
  Byte_01 : Constant  Value=char(2, E)  OutDataTypeStr=uint8
  Byte_02 : Constant  Value=char(3, E)  OutDataTypeStr=uint8
  Byte_03 : Constant  Value=char(4, E)  OutDataTypeStr=uint8
  Byte_04 : Constant  Value=char(5, E)  OutDataTypeStr=uint8
  Byte_05 : Constant  Value=char(6, E)  OutDataTypeStr=uint8
  Byte_06 : Constant  Value=char(7, E)  OutDataTypeStr=uint8
  Byte_07 : Constant  Value=char(8, E)  OutDataTypeStr=uint8
  Byte_1 : Constant  Value=char(1, E)  OutDataTypeStr=uint8
  Column_1(1B) : Outport
  Column_2(1B) : Outport  Port=2
  Column_3(1B) : Outport  Port=3
  Column_4(1B) : Outport  Port=4
  Column_5(1B) : Outport  Port=5
  Column_6(1B) : Outport  Port=6
  Column_7(1B) : Outport  Port=7
  Column_8(1B) : Outport  Port=8
  wires:
  Byte_05/1 -> Column_6(1B)/1
  Byte_04/1 -> Column_5(1B)/1
  Byte_01/1 -> Column_2(1B)/1
  Byte_07/1 -> Column_8(1B)/1
  Byte_03/1 -> Column_4(1B)/1
  Byte_06/1 -> Column_7(1B)/1
  Byte_1/1 -> Column_1(1B)/1
  Byte_02/1 -> Column_3(1B)/1

== system Computer_Library/Character_Table/Characters(0..F)/Char_F ==
  Byte_01 : Constant  Value=char(2, F)  OutDataTypeStr=uint8
  Byte_02 : Constant  Value=char(3, F)  OutDataTypeStr=uint8
  Byte_03 : Constant  Value=char(4, F)  OutDataTypeStr=uint8
  Byte_04 : Constant  Value=char(5, F)  OutDataTypeStr=uint8
  Byte_05 : Constant  Value=char(6, F)  OutDataTypeStr=uint8
  Byte_06 : Constant  Value=char(7, F)  OutDataTypeStr=uint8
  Byte_07 : Constant  Value=char(8, F)  OutDataTypeStr=uint8
  Byte_1 : Constant  Value=char(1, F)  OutDataTypeStr=uint8
  Column_1(1B) : Outport
  Column_2(1B) : Outport  Port=2
  Column_3(1B) : Outport  Port=3
  Column_4(1B) : Outport  Port=4
  Column_5(1B) : Outport  Port=5
  Column_6(1B) : Outport  Port=6
  Column_7(1B) : Outport  Port=7
  Column_8(1B) : Outport  Port=8
  wires:
  Byte_05/1 -> Column_6(1B)/1
  Byte_04/1 -> Column_5(1B)/1
  Byte_01/1 -> Column_2(1B)/1
  Byte_07/1 -> Column_8(1B)/1
  Byte_03/1 -> Column_4(1B)/1
  Byte_06/1 -> Column_7(1B)/1
  Byte_1/1 -> Column_1(1B)/1
  Byte_02/1 -> Column_3(1B)/1

== system Computer_Library/Character_Table/Characters(ARROW_DOWN..RECTANGLE)/Char_ARROW_DOWN ==
  Byte_01 : Constant  Value=char(2, ARROW_DOWN)  OutDataTypeStr=uint8
  Byte_02 : Constant  Value=char(3, ARROW_DOWN)  OutDataTypeStr=uint8
  Byte_03 : Constant  Value=char(4, ARROW_DOWN)  OutDataTypeStr=uint8
  Byte_04 : Constant  Value=char(5, ARROW_DOWN)  OutDataTypeStr=uint8
  Byte_05 : Constant  Value=char(6, ARROW_DOWN)  OutDataTypeStr=uint8
  Byte_06 : Constant  Value=char(7, ARROW_DOWN)  OutDataTypeStr=uint8
  Byte_07 : Constant  Value=char(8, ARROW_DOWN)  OutDataTypeStr=uint8
  Byte_1 : Constant  Value=char(1, ARROW_DOWN)  OutDataTypeStr=uint8
  Column_1(1B) : Outport
  Column_2(1B) : Outport  Port=2
  Column_3(1B) : Outport  Port=3
  Column_4(1B) : Outport  Port=4
  Column_5(1B) : Outport  Port=5
  Column_6(1B) : Outport  Port=6
  Column_7(1B) : Outport  Port=7
  Column_8(1B) : Outport  Port=8
  wires:
  Byte_05/1 -> Column_6(1B)/1
  Byte_04/1 -> Column_5(1B)/1
  Byte_01/1 -> Column_2(1B)/1
  Byte_07/1 -> Column_8(1B)/1
  Byte_03/1 -> Column_4(1B)/1
  Byte_06/1 -> Column_7(1B)/1
  Byte_1/1 -> Column_1(1B)/1
  Byte_02/1 -> Column_3(1B)/1

== system Computer_Library/Character_Table/Characters(ARROW_DOWN..RECTANGLE)/Char_ARROW_LEFT ==
  Byte_01 : Constant  Value=char(2, ARROW_LEFT)  OutDataTypeStr=uint8
  Byte_02 : Constant  Value=char(3, ARROW_LEFT)  OutDataTypeStr=uint8
  Byte_03 : Constant  Value=char(4, ARROW_LEFT)  OutDataTypeStr=uint8
  Byte_04 : Constant  Value=char(5, ARROW_LEFT)  OutDataTypeStr=uint8
  Byte_05 : Constant  Value=char(6, ARROW_LEFT)  OutDataTypeStr=uint8
  Byte_06 : Constant  Value=char(7, ARROW_LEFT)  OutDataTypeStr=uint8
  Byte_07 : Constant  Value=char(8, ARROW_LEFT)  OutDataTypeStr=uint8
  Byte_1 : Constant  Value=char(1, ARROW_LEFT)  OutDataTypeStr=uint8
  Column_1(1B) : Outport
  Column_2(1B) : Outport  Port=2
  Column_3(1B) : Outport  Port=3
  Column_4(1B) : Outport  Port=4
  Column_5(1B) : Outport  Port=5
  Column_6(1B) : Outport  Port=6
  Column_7(1B) : Outport  Port=7
  Column_8(1B) : Outport  Port=8
  wires:
  Byte_05/1 -> Column_6(1B)/1
  Byte_04/1 -> Column_5(1B)/1
  Byte_01/1 -> Column_2(1B)/1
  Byte_07/1 -> Column_8(1B)/1
  Byte_03/1 -> Column_4(1B)/1
  Byte_06/1 -> Column_7(1B)/1
  Byte_1/1 -> Column_1(1B)/1
  Byte_02/1 -> Column_3(1B)/1

== system Computer_Library/Character_Table/Characters(ARROW_DOWN..RECTANGLE)/Char_ARROW_RIGHT ==
  Byte_01 : Constant  Value=char(2, ARROW_RIGHT)  OutDataTypeStr=uint8
  Byte_02 : Constant  Value=char(3, ARROW_RIGHT)  OutDataTypeStr=uint8
  Byte_03 : Constant  Value=char(4, ARROW_RIGHT)  OutDataTypeStr=uint8
  Byte_04 : Constant  Value=char(5, ARROW_RIGHT)  OutDataTypeStr=uint8
  Byte_05 : Constant  Value=char(6, ARROW_RIGHT)  OutDataTypeStr=uint8
  Byte_06 : Constant  Value=char(7, ARROW_RIGHT)  OutDataTypeStr=uint8
  Byte_07 : Constant  Value=char(8, ARROW_RIGHT)  OutDataTypeStr=uint8
  Byte_1 : Constant  Value=char(1, ARROW_RIGHT)  OutDataTypeStr=uint8
  Column_1(1B) : Outport
  Column_2(1B) : Outport  Port=2
  Column_3(1B) : Outport  Port=3
  Column_4(1B) : Outport  Port=4
  Column_5(1B) : Outport  Port=5
  Column_6(1B) : Outport  Port=6
  Column_7(1B) : Outport  Port=7
  Column_8(1B) : Outport  Port=8
  wires:
  Byte_05/1 -> Column_6(1B)/1
  Byte_04/1 -> Column_5(1B)/1
  Byte_01/1 -> Column_2(1B)/1
  Byte_07/1 -> Column_8(1B)/1
  Byte_03/1 -> Column_4(1B)/1
  Byte_06/1 -> Column_7(1B)/1
  Byte_1/1 -> Column_1(1B)/1
  Byte_02/1 -> Column_3(1B)/1

== system Computer_Library/Character_Table/Characters(ARROW_DOWN..RECTANGLE)/Char_COMMA ==
  Byte_01 : Constant  Value=char(2, COMMA)  OutDataTypeStr=uint8
  Byte_02 : Constant  Value=char(3, COMMA)  OutDataTypeStr=uint8
  Byte_03 : Constant  Value=char(4, COMMA)  OutDataTypeStr=uint8
  Byte_04 : Constant  Value=char(5, COMMA)  OutDataTypeStr=uint8
  Byte_05 : Constant  Value=char(6, COMMA)  OutDataTypeStr=uint8
  Byte_06 : Constant  Value=char(7, COMMA)  OutDataTypeStr=uint8
  Byte_07 : Constant  Value=char(8, COMMA)  OutDataTypeStr=uint8
  Byte_1 : Constant  Value=char(1, COMMA)  OutDataTypeStr=uint8
  Column_1(1B) : Outport
  Column_2(1B) : Outport  Port=2
  Column_3(1B) : Outport  Port=3
  Column_4(1B) : Outport  Port=4
  Column_5(1B) : Outport  Port=5
  Column_6(1B) : Outport  Port=6
  Column_7(1B) : Outport  Port=7
  Column_8(1B) : Outport  Port=8
  wires:
  Byte_05/1 -> Column_6(1B)/1
  Byte_04/1 -> Column_5(1B)/1
  Byte_01/1 -> Column_2(1B)/1
  Byte_07/1 -> Column_8(1B)/1
  Byte_03/1 -> Column_4(1B)/1
  Byte_06/1 -> Column_7(1B)/1
  Byte_1/1 -> Column_1(1B)/1
  Byte_02/1 -> Column_3(1B)/1

== system Computer_Library/Character_Table/Characters(ARROW_DOWN..RECTANGLE)/Char_CURSOR ==
  Byte_01 : Constant  Value=char(2, CURSOR)  OutDataTypeStr=uint8
  Byte_02 : Constant  Value=char(3, CURSOR)  OutDataTypeStr=uint8
  Byte_03 : Constant  Value=char(4, CURSOR)  OutDataTypeStr=uint8
  Byte_04 : Constant  Value=char(5, CURSOR)  OutDataTypeStr=uint8
  Byte_05 : Constant  Value=char(6, CURSOR)  OutDataTypeStr=uint8
  Byte_06 : Constant  Value=char(7, CURSOR)  OutDataTypeStr=uint8
  Byte_07 : Constant  Value=char(8, CURSOR)  OutDataTypeStr=uint8
  Byte_1 : Constant  Value=char(1, CURSOR)  OutDataTypeStr=uint8
  Column_1(1B) : Outport
  Column_2(1B) : Outport  Port=2
  Column_3(1B) : Outport  Port=3
  Column_4(1B) : Outport  Port=4
  Column_5(1B) : Outport  Port=5
  Column_6(1B) : Outport  Port=6
  Column_7(1B) : Outport  Port=7
  Column_8(1B) : Outport  Port=8
  wires:
  Byte_05/1 -> Column_6(1B)/1
  Byte_04/1 -> Column_5(1B)/1
  Byte_01/1 -> Column_2(1B)/1
  Byte_07/1 -> Column_8(1B)/1
  Byte_03/1 -> Column_4(1B)/1
  Byte_06/1 -> Column_7(1B)/1
  Byte_1/1 -> Column_1(1B)/1
  Byte_02/1 -> Column_3(1B)/1

== system Computer_Library/Character_Table/Characters(ARROW_DOWN..RECTANGLE)/Char_DOT ==
  Byte_01 : Constant  Value=char(2, DOT)  OutDataTypeStr=uint8
  Byte_02 : Constant  Value=char(3, DOT)  OutDataTypeStr=uint8
  Byte_03 : Constant  Value=char(4, DOT)  OutDataTypeStr=uint8
  Byte_04 : Constant  Value=char(5, DOT)  OutDataTypeStr=uint8
  Byte_05 : Constant  Value=char(6, DOT)  OutDataTypeStr=uint8
  Byte_06 : Constant  Value=char(7, DOT)  OutDataTypeStr=uint8
  Byte_07 : Constant  Value=char(8, DOT)  OutDataTypeStr=uint8
  Byte_1 : Constant  Value=char(1, DOT)  OutDataTypeStr=uint8
  Column_1(1B) : Outport
  Column_2(1B) : Outport  Port=2
  Column_3(1B) : Outport  Port=3
  Column_4(1B) : Outport  Port=4
  Column_5(1B) : Outport  Port=5
  Column_6(1B) : Outport  Port=6
  Column_7(1B) : Outport  Port=7
  Column_8(1B) : Outport  Port=8
  wires:
  Byte_05/1 -> Column_6(1B)/1
  Byte_04/1 -> Column_5(1B)/1
  Byte_01/1 -> Column_2(1B)/1
  Byte_07/1 -> Column_8(1B)/1
  Byte_03/1 -> Column_4(1B)/1
  Byte_06/1 -> Column_7(1B)/1
  Byte_1/1 -> Column_1(1B)/1
  Byte_02/1 -> Column_3(1B)/1

== system Computer_Library/Character_Table/Characters(ARROW_DOWN..RECTANGLE)/Char_EXCLAMATION_MARK ==
  Byte_01 : Constant  Value=char(2, EXCLAMATION_MARK)  OutDataTypeStr=uint8
  Byte_02 : Constant  Value=char(3, EXCLAMATION_MARK)  OutDataTypeStr=uint8
  Byte_03 : Constant  Value=char(4, EXCLAMATION_MARK)  OutDataTypeStr=uint8
  Byte_04 : Constant  Value=char(5, EXCLAMATION_MARK)  OutDataTypeStr=uint8
  Byte_05 : Constant  Value=char(6, EXCLAMATION_MARK)  OutDataTypeStr=uint8
  Byte_06 : Constant  Value=char(7, EXCLAMATION_MARK)  OutDataTypeStr=uint8
  Byte_07 : Constant  Value=char(8, EXCLAMATION_MARK)  OutDataTypeStr=uint8
  Byte_1 : Constant  Value=char(1, EXCLAMATION_MARK)  OutDataTypeStr=uint8
  Column_1(1B) : Outport
  Column_2(1B) : Outport  Port=2
  Column_3(1B) : Outport  Port=3
  Column_4(1B) : Outport  Port=4
  Column_5(1B) : Outport  Port=5
  Column_6(1B) : Outport  Port=6
  Column_7(1B) : Outport  Port=7
  Column_8(1B) : Outport  Port=8
  wires:
  Byte_05/1 -> Column_6(1B)/1
  Byte_04/1 -> Column_5(1B)/1
  Byte_01/1 -> Column_2(1B)/1
  Byte_07/1 -> Column_8(1B)/1
  Byte_03/1 -> Column_4(1B)/1
  Byte_06/1 -> Column_7(1B)/1
  Byte_1/1 -> Column_1(1B)/1
  Byte_02/1 -> Column_3(1B)/1

== system Computer_Library/Character_Table/Characters(ARROW_DOWN..RECTANGLE)/Char_LEFT_PARENTHESES ==
  Byte_01 : Constant  Value=char(2, LEFT_PARENTHESES)  OutDataTypeStr=uint8
  Byte_02 : Constant  Value=char(3, LEFT_PARENTHESES)  OutDataTypeStr=uint8
  Byte_03 : Constant  Value=char(4, LEFT_PARENTHESES)  OutDataTypeStr=uint8
  Byte_04 : Constant  Value=char(5, LEFT_PARENTHESES)  OutDataTypeStr=uint8
  Byte_05 : Constant  Value=char(6, LEFT_PARENTHESES)  OutDataTypeStr=uint8
  Byte_06 : Constant  Value=char(7, LEFT_PARENTHESES)  OutDataTypeStr=uint8
  Byte_07 : Constant  Value=char(8, LEFT_PARENTHESES)  OutDataTypeStr=uint8
  Byte_1 : Constant  Value=char(1, LEFT_PARENTHESES)  OutDataTypeStr=uint8
  Column_1(1B) : Outport
  Column_2(1B) : Outport  Port=2
  Column_3(1B) : Outport  Port=3
  Column_4(1B) : Outport  Port=4
  Column_5(1B) : Outport  Port=5
  Column_6(1B) : Outport  Port=6
  Column_7(1B) : Outport  Port=7
  Column_8(1B) : Outport  Port=8
  wires:
  Byte_05/1 -> Column_6(1B)/1
  Byte_04/1 -> Column_5(1B)/1
  Byte_01/1 -> Column_2(1B)/1
  Byte_07/1 -> Column_8(1B)/1
  Byte_03/1 -> Column_4(1B)/1
  Byte_06/1 -> Column_7(1B)/1
  Byte_1/1 -> Column_1(1B)/1
  Byte_02/1 -> Column_3(1B)/1

== system Computer_Library/Character_Table/Characters(ARROW_DOWN..RECTANGLE)/Char_PERCENT ==
  Byte_01 : Constant  Value=char(2, PERCENT)  OutDataTypeStr=uint8
  Byte_02 : Constant  Value=char(3, PERCENT)  OutDataTypeStr=uint8
  Byte_03 : Constant  Value=char(4, PERCENT)  OutDataTypeStr=uint8
  Byte_04 : Constant  Value=char(5, PERCENT)  OutDataTypeStr=uint8
  Byte_05 : Constant  Value=char(6, PERCENT)  OutDataTypeStr=uint8
  Byte_06 : Constant  Value=char(7, PERCENT)  OutDataTypeStr=uint8
  Byte_07 : Constant  Value=char(8, PERCENT)  OutDataTypeStr=uint8
  Byte_1 : Constant  Value=char(1, PERCENT)  OutDataTypeStr=uint8
  Column_1(1B) : Outport
  Column_2(1B) : Outport  Port=2
  Column_3(1B) : Outport  Port=3
  Column_4(1B) : Outport  Port=4
  Column_5(1B) : Outport  Port=5
  Column_6(1B) : Outport  Port=6
  Column_7(1B) : Outport  Port=7
  Column_8(1B) : Outport  Port=8
  wires:
  Byte_05/1 -> Column_6(1B)/1
  Byte_04/1 -> Column_5(1B)/1
  Byte_01/1 -> Column_2(1B)/1
  Byte_07/1 -> Column_8(1B)/1
  Byte_03/1 -> Column_4(1B)/1
  Byte_06/1 -> Column_7(1B)/1
  Byte_1/1 -> Column_1(1B)/1
  Byte_02/1 -> Column_3(1B)/1

== system Computer_Library/Character_Table/Characters(ARROW_DOWN..RECTANGLE)/Char_QUESTION_MARK ==
  Byte_01 : Constant  Value=char(2, QUESTION_MARK)  OutDataTypeStr=uint8
  Byte_02 : Constant  Value=char(3, QUESTION_MARK)  OutDataTypeStr=uint8
  Byte_03 : Constant  Value=char(4, QUESTION_MARK)  OutDataTypeStr=uint8
  Byte_04 : Constant  Value=char(5, QUESTION_MARK)  OutDataTypeStr=uint8
  Byte_05 : Constant  Value=char(6, QUESTION_MARK)  OutDataTypeStr=uint8
  Byte_06 : Constant  Value=char(7, QUESTION_MARK)  OutDataTypeStr=uint8
  Byte_07 : Constant  Value=char(8, QUESTION_MARK)  OutDataTypeStr=uint8
  Byte_1 : Constant  Value=char(1, QUESTION_MARK)  OutDataTypeStr=uint8
  Column_1(1B) : Outport
  Column_2(1B) : Outport  Port=2
  Column_3(1B) : Outport  Port=3
  Column_4(1B) : Outport  Port=4
  Column_5(1B) : Outport  Port=5
  Column_6(1B) : Outport  Port=6
  Column_7(1B) : Outport  Port=7
  Column_8(1B) : Outport  Port=8
  wires:
  Byte_05/1 -> Column_6(1B)/1
  Byte_04/1 -> Column_5(1B)/1
  Byte_01/1 -> Column_2(1B)/1
  Byte_07/1 -> Column_8(1B)/1
  Byte_03/1 -> Column_4(1B)/1
  Byte_06/1 -> Column_7(1B)/1
  Byte_1/1 -> Column_1(1B)/1
  Byte_02/1 -> Column_3(1B)/1
